simulink model "ArduCopter_MinnieLoiterFtc"  (R2018b)
settings: Solver=FixedStepDiscrete  StartTime=0.0  StopTime=1000  FixedStep=cntrl.sample_time  RelTol=1e-4
libraries: simulink x3, ardupilot_custom_controller_lib x2, copterFtc_lib x2, axes_transformation_lib x1
settings Model: DataTypeOverride=Single  DataTypeOverrideAppliesTo=Floating-point  Creator=Yannic  LastModifiedBy=yannic
settings SolverCC: ZeroCrossControl=DisableAll
settings DataIOCC: LimitDataPoints=on  SaveOutput=off  SaveTime=off  ReturnWorkspaceOutputs=on
settings OptimizationCC: DefaultParameterBehavior=Inlined  UseFloatMulNetSlope=on  DefaultUnderspecifiedDataType=single  InlineInvariantSignals=on  PassReuseOutputArgsAs=Individual arguments  ZeroExternalMemoryAtStartup=off  ZeroInternalMemoryAtStartup=off  NoFixptDivByZeroProtection=on  EfficientFloat2IntCast=on  LifeSpan=1  OptimizeBlockOrder=speed  DifferentSizesBufferReuse=on
settings DebuggingCC: ReadBeforeWriteMsg=DisableAll  WriteAfterWriteMsg=DisableAll  WriteAfterReadMsg=DisableAll  MultiTaskDSMMsg=none  ParameterTunabilityLossMsg=error  AllowSymbolicDim=off  LibraryContextMissingDiagnostic=none  SFUnexpectedBacktrackingDiag=warning  SFNoUnconditionalDefaultTransitionDiag=warning  SFExecutionAtInitializationDiag=none
settings HardwareCC: ProdBitPerPointer=32  ProdBitPerSizeT=32  ProdBitPerPtrDiffT=32  ProdLargestAtomicInteger=Long  ProdWordSize=32  ProdHWDeviceType=ARM Compatible->ARM 7
settings ModelReferenceCC: UpdateModelReferenceTargets=IfOutOfDate  PropagateSignalLabelsOutOfModel=off
settings SFSimCC: SFSimEcho=off  SimUseLocalCustomCode=off  MATLABDynamicMemAlloc=off
settings RTWCC: SystemTargetFile=ert.tlc  GenCodeOnly=on  TemplateMakefile=ert_default_tmf  GenerateReport=on  RTWUseLocalCustomCode=off  IncludeHyperlinkInReport=on  LaunchReport=on  TargetLang=C++  GenerateTraceInfo=on  GenerateTraceReport=on  GenerateTraceReportSl=on  GenerateTraceReportSf=on  GenerateTraceReportEml=on
settings CodeAppCC: ForceParamTrailComments=on  IgnoreCustomStorageClasses=off  OperatorAnnotations=on  SimulinkDataObjDesc=on  SFDataObjDesc=on  CustomSymbolStrGlobalVar=rt$N$M  CustomSymbolStrType=$N$M  CustomSymbolStrFcn=$N$M$F  CustomSymbolStrMacro=$N$M  InsertBlockDesc=on
settings ERTTargetCC: TargetLangStandard=C++03 (ISO)  GenerateSampleERTMain=on  IncludeMdlTerminateFcn=off  CombineSignalStateStructs=on  SuppressErrorStatus=on  SupportAbsoluteTime=off  MultiInstanceERTCode=on  CodeInterfacePackaging=C++ class  SupportNonFinite=off  SupportComplex=off  SupportVariableSizeSignals=on  ERTHeaderFileRootName=MatlabController$E  ERTSourceFileRootName=MatlabController$E  ERTDataFileRootName=MatlabController_data  InlinedParameterPlacement=NonHierarchical  RootIOFormat=Structure reference  ERTCustomFileTemplate=example_file_process.tlc  ERTFilePackagingFormat=CompactWithDataFile
settings ConfigComp: CovMetricSettings=dw  CovHtmlReporting=on  CovSaveCumulativeToWorkspaceVar=on  CovSaveSingleToWorkspaceVar=on  CovExternalEMLEnable=off

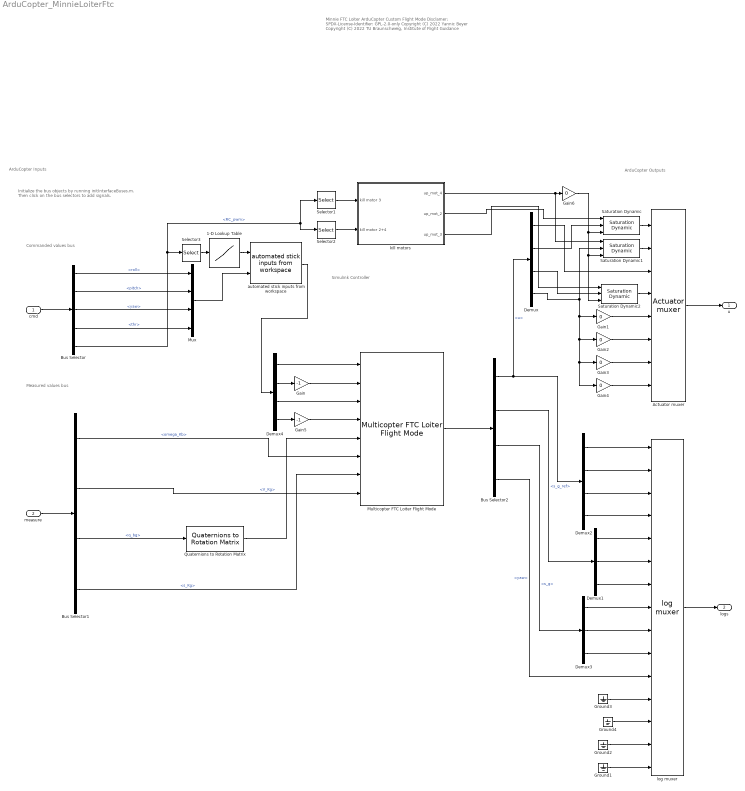
== system ArduCopter_MinnieLoiterFtc ==
  note: Measured values bus
  note: Initialize the bus objects by running initInterfaceBuses.m.
      | Then click on the bus selectors to add signals.
  note: Commanded values bus
  note: ArduCopter Inputs
  note: ArduCopter Outputs
  note: Simulink Controller
  note: Minnie FTC Loiter ArduCopter Custom Flight Mode
      |
      | Disclamer:
      | SPDX-License-Identifier: GPL-2.0-only
      |
      | Copyright (C) 2022 Yannic Beyer
      | Copyright (C) 2022 TU Braunschweig, Institute of Flight Guidance
  cmd : Inport  OutDataTypeStr=Bus: cmdBus
  measure : Inport  Port=2  OutDataTypeStr=Bus: measureBus
  1-D Lookup Table : Lookup_n-D  NumberOfTableDimensions=1  BreakpointsForDimension1=[1000;2000]  Table=[0;1]  InternalRulePriority=Speed  RndMeth=Simplest  InputSameDT=on
  Actuator muxer : ardupilot_custom_controller_lib/Actuator muxer
      settings: SourceProductName=LADAC
  Bus Selector : BusSelector  OutputSignals=roll,pitch,yaw,thr,RC_pwm
  Bus Selector1 : BusSelector  OutputSignals=omega_Kb,V_Kg,q_bg,s_Kg
  Bus Selector2 : BusSelector  OutputSignals=u,pos_cntrl.reference.s_g_ref,pos_cntrl.measure.s_g,atti_cntrl.measure.yaw
  Demux : Demux
  Demux1 : Demux  Outputs=3
  Demux2 : Demux
  Demux3 : Demux  Outputs=3
  Demux4 : Demux
  Gain : Gain  Gain=-1
  Gain{1..4,6} (5 alike) : Gain  Gain=0
  Gain5 : Gain  Gain=-1
  Ground{1..4} (4 alike) : Ground
  Multicopter FTC Loiter Flight Mode : copterFtc_lib/Multicopter FTC Loiter Flight Mode  fm=fm_loiter
      settings: SourceProductName=Copter FTC
  Mux : Mux
  Quaternions to Rotation Matrix : axes_transformation_lib/Quaternions to Rotation Matrix  SystemSampleTime=-1
      settings: SourceProductName=LADAC
  Saturation Dynamic : simulink/Discontinuities/Saturation Dynamic  OutMin=[]  OutMax=[]  OutDataTypeStr=Inherit: Same as second input  OutDataType=fixdt(1, 16)  OutScaling=2^-10  DoSatur=off
  Saturation Dynamic1 : simulink/Discontinuities/Saturation Dynamic  OutMin=[]  OutMax=[]  OutDataTypeStr=Inherit: Same as second input  OutDataType=fixdt(1, 16)  OutScaling=2^-10  DoSatur=off
  Saturation Dynamic2 : simulink/Discontinuities/Saturation Dynamic  OutMin=[]  OutMax=[]  OutDataTypeStr=Inherit: Same as second input  OutDataType=fixdt(1, 16)  OutScaling=2^-10  DoSatur=off
  Selector1 : Selector  InputPortWidth=16  IndexOptions=Index vector (dialog)  Indices=7  OutputSizes=1
  Selector2 : Selector  InputPortWidth=16  IndexOptions=Index vector (dialog)  Indices=8  OutputSizes=1
  Selector3 : Selector  InputPortWidth=16  IndexOptions=Index vector (dialog)  Indices=9  OutputSizes=1
  automated stick inputs from workspace : copterFtc_lib/automated stick inputs from workspace  simin=simin
      settings: SourceProductName=Copter FTC
  kill motors : Subsystem
  log muxer : ardupilot_custom_controller_lib/log muxer
      settings: SourceProductName=LADAC
  u : Outport
  logs : Outport  Port=2
  wires:
  cmd/1 -> Bus Selector/1
  measure/1 -> Bus Selector1/1
  Bus Selector/1 -> Mux/1  "<roll>"
  Bus Selector/2 -> Mux/2  "<pitch>"
  Bus Selector/3 -> Mux/3  "<yaw>"
  Bus Selector/4 -> Mux/4  "<thr>"
  Actuator muxer/1 -> u/1
  log muxer/1 -> logs/1
  Ground1/1 -> log muxer/15
  Selector2/1 -> kill motors/2(kill motor 2+4)
  Bus Selector/5 -> Selector1/1, Selector2/1, Selector3/1  "<RC_pwm>"
  Selector1/1 -> kill motors/1(kill motor 3)
  Demux/4 -> Saturation Dynamic1/2, Gain1/1, Gain4/1, Gain3/1, Gain2/1
  Multicopter FTC Loiter Flight Mode/1 -> Bus Selector2/1
  Demux3/2 -> log muxer/9
  Demux/3 -> Saturation Dynamic2/2
  Demux1/1 -> log muxer/5
  kill motors/3(up_mot_3) -> Saturation Dynamic2/1
  kill motors/2(up_mot_2) -> Saturation Dynamic/1
  Gain1/1 -> Actuator muxer/5
  Gain4/1 -> Actuator muxer/8
  Demux1/3 -> log muxer/7
  Demux1/2 -> log muxer/6
  Gain3/1 -> Actuator muxer/7
  Demux2/2 -> log muxer/2
  Bus Selector2/1 -> Demux/1, Demux2/1  "<u>"
  Demux/2 -> Saturation Dynamic/2
  kill motors/1(up_mot_4) -> Gain6/1, Saturation Dynamic1/1
  Demux2/3 -> log muxer/3
  Demux3/1 -> log muxer/8
  Gain2/1 -> Actuator muxer/6
  Demux/1 -> Actuator muxer/3
  Gain6/1 -> Saturation Dynamic/3, Saturation Dynamic1/3, Saturation Dynamic2/3
  Demux2/4 -> log muxer/4
  Demux2/1 -> log muxer/1
  Saturation Dynamic/1 -> Actuator muxer/1
  Saturation Dynamic1/1 -> Actuator muxer/2
  Saturation Dynamic2/1 -> Actuator muxer/4
  Demux3/3 -> log muxer/10
  Bus Selector2/4 -> log muxer/11  "<yaw>"
  Ground3/1 -> log muxer/12
  Ground4/1 -> log muxer/13
  Ground2/1 -> log muxer/14
  Bus Selector1/1 -> Multicopter FTC Loiter Flight Mode/6  "<omega_Kb>"
  Bus Selector1/2 -> Multicopter FTC Loiter Flight Mode/8  "<V_Kg>"
  Bus Selector1/3 -> Quaternions to Rotation Matrix/1  "<q_bg>"
  Quaternions to Rotation Matrix/1 -> Multicopter FTC Loiter Flight Mode/5
  Bus Selector1/4 -> Multicopter FTC Loiter Flight Mode/7  "<s_Kg>"
  Gain/1 -> Multicopter FTC Loiter Flight Mode/2
  Gain5/1 -> Multicopter FTC Loiter Flight Mode/4
  Bus Selector2/2 -> Demux1/1  "<s_g_ref>"
  Bus Selector2/3 -> Demux3/1  "<s_g>"
  Selector3/1 -> 1-D Lookup Table/1
  1-D Lookup Table/1 -> automated stick inputs from workspace/1
  Mux/1 -> automated stick inputs from workspace/2
  Demux4/2 -> Gain/1
  Demux4/4 -> Gain5/1
  Demux4/3 -> Multicopter FTC Loiter Flight Mode/3
  Demux4/1 -> Multicopter FTC Loiter Flight Mode/1
  automated stick inputs from workspace/1 -> Demux4/1

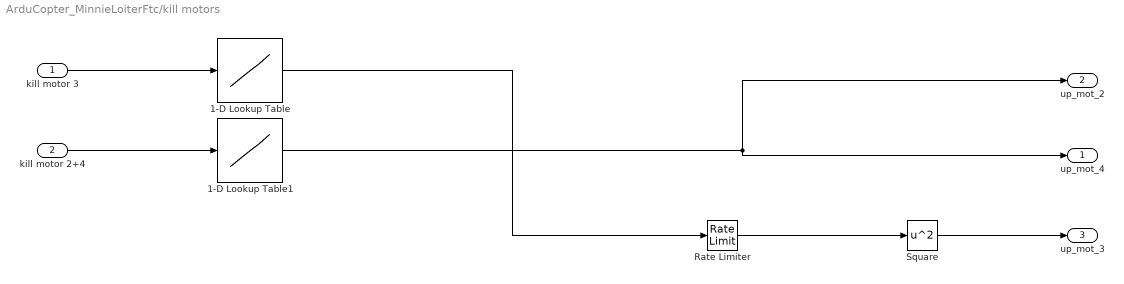
== system ArduCopter_MinnieLoiterFtc/kill motors ==
  kill motor 3 : Inport
  kill motor 2+4 : Inport  Port=2
  1-D Lookup Table : Lookup_n-D  NumberOfTableDimensions=1  BreakpointsForDimension1=[1000;2000]  Table=[1;0.1]  InternalRulePriority=Speed  RndMeth=Simplest  InputSameDT=on
  1-D Lookup Table1 : Lookup_n-D  NumberOfTableDimensions=1  BreakpointsForDimension1=[1000;2000]  Table=[1;0.1]  InternalRulePriority=Speed  RndMeth=Simplest  InputSameDT=on
  Rate Limiter : RateLimiter  RisingSlewLimit=1000  FallingSlewLimit=-0.1  SampleTimeMode=inherited
  Square : Math  Operator=square  SaturateOnIntegerOverflow=on
  up_mot_4 : Outport
  up_mot_2 : Outport  Port=2
  up_mot_3 : Outport  Port=3
  wires:
  1-D Lookup Table1/1 -> up_mot_2/1, up_mot_4/1
  kill motor 3/1 -> 1-D Lookup Table/1
  kill motor 2+4/1 -> 1-D Lookup Table1/1
  1-D Lookup Table/1 -> Rate Limiter/1
  Rate Limiter/1 -> Square/1
  Square/1 -> up_mot_3/1
